simulink model "rasberry"  (R2016b)
settings: Solver=VariableStepAuto  StartTime=0.0  StopTime=10.0  RelTol=1e-3
libraries: embdlinuxlib x1
settings Model: Creator=sbuadu  LastModifiedBy=sbuadu

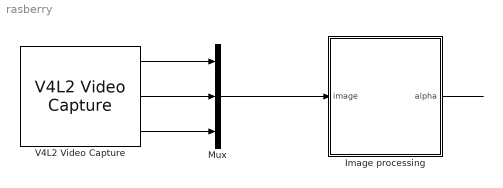
== system rasberry ==
  Image processing : Subsystem
  Mux : Mux  Inputs=3
  V4L2 Video Capture : embdlinuxlib/V4L2 Video Capture  m_devName='/dev/video0'  roi=[0, 0, 640, 480]  imSizeSelection=160x120  imSize=[640, 480]  pixelFormat=RGB  pixelOrder=Planar  sampleTime=1/10  simOutput=Colorbars  blockPlatform=Raspberry Pi
  wires:
  V4L2 Video Capture/1 -> Mux/1
  V4L2 Video Capture/2 -> Mux/2
  V4L2 Video Capture/3 -> Mux/3
  Mux/1 -> Image processing/1("image ")
  Image processing/1(alpha) -> ?

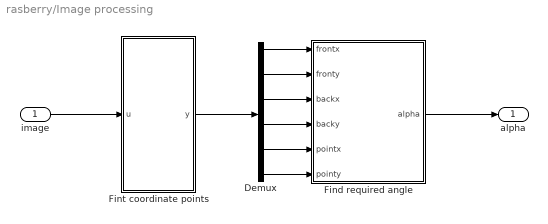
== system rasberry/Image processing ==
  "image " : Inport
  Demux : Demux  Outputs=6
  Find required angle : MATLAB Function  TreatAsAtomicUnit=on
  Fint coordinate points : MATLAB Function  TreatAsAtomicUnit=on
  alpha : Outport
  wires:
  Demux/2 -> Find required angle/2(fronty)
  Demux/4 -> Find required angle/4(backy)
  Demux/1 -> Find required angle/1(frontx)
  Demux/3 -> Find required angle/3(backx)
  Demux/5 -> Find required angle/5(pointx)
  Demux/6 -> Find required angle/6(pointy)
  "image "/1 -> Fint coordinate points/1(u)
  Find required angle/1(alpha) -> alpha/1
  Fint coordinate points/1(y) -> Demux/1

== matlab function rasberry/Image processing/Fint coordinate points ==
  data: u input; y output
function y = fcn(u)

y = u;

== matlab function rasberry/Image processing/Find required angle ==
  data: frontx input; alpha output; fronty input; backx input; backy input; pointx input; pointy input
function alpha =  findAngle(frontx, fronty, backx, backy, pointx, pointy)

%%setting the coordinates for the middle of the car 
if frontx < backx
    carx = frontx + abs(backx - frontx)/2; 
else
    carx = backx + abs(backx - frontx)/2; 
end

if fronty < backy
    cary = fronty + abs(backy - fronty)/2; 
else
    cary = backy + abs(backy - fronty)/2;  
end


%%finding the vector between car and destination 
deltax = pointx - carx; 
deltay = pointy-cary; 
delta = [deltax deltay]; 
%%tvector from rotation point to frot of vehicle
betax = frontx - carx;
betay = fronty-cary; 
beta = [betax betay]; 

alpha = atan2(beta(2), beta(1)) - atan2(delta(2), delta(1)); 

alpha = alpha*180/pi; 

if alpha > 180
alpha = alpha - 360; 
end


end
